simulink model "e5_3blocks_nn"  (R2020a)
settings: Solver=VariableStepAuto  StartTime=0.0  StopTime=10.0  RelTol=1e-3
undefined symbols (not defined in the file or in its folder): Quad
libraries: neural x123
(part 6 of 6)

== system e5_3blocks_nn/NN_online/Layer 3/Delays 1 ==
  "p{3}" : Inport  PortDimensions=30
      mask Display: e = 0.06;c1 = [120 230 180]/255;c2 = ([120 230 180]+0)/(256+128);c3 = ([120 230 180]+128)/(256+128);patch([0 1 1 0],[0 0 1 1],c1);patch([0 1 1 1-e 1-e 0+e],[0 0 1 1-e 0+e 0+e],c2);patch([0 0 1 1-e 0+e 0+e],[0 1 1 1-e 1-e 0+e],c3);plot([0 1 1 0 0],[0 0 1 1 0]);
  mux : Mux  Inputs=1
      mask Display: e = 0.06;c1 = [120 150 230]/255;c2 = ([120 150 230]+0)/383;c3 = ([120 150 230]+128)/383;patch([0 1 1 0],[0 0 1 1],c1);patch([0 1 1 1-e 1-e 0+e],[0 0 1 1-e 0+e 0+e],c2);patch([0 0 1 1-e 0+e 0+e],[0 1 1 1-e 1-e 0+e],c3);plot([0 1 1 0 0],[0 0 1 1 0]);disp('Mux')
  "pd{3,2}" : Outport
      mask Display: e = 0.06;c1 = [120 230 180]/255;c2 = ([120 230 180]+0)/(256+128);c3 = ([120 230 180]+128)/(256+128);patch([0 1 1 0],[0 0 1 1],c1);patch([0 1 1 1-e 1-e 0+e],[0 0 1 1-e 0+e 0+e],c2);patch([0 0 1 1-e 0+e 0+e],[0 1 1 1-e 1-e 0+e],c3);plot([0 1 1 0 0],[0 0 1 1 0]);
  wires:
  "p{3}"/1 -> mux/1
  mux/1 -> "pd{3,2}"/1

== system e5_3blocks_nn/NN_online/Layer 3/LW{3,2} ==
  "ad{3,2}" : Inport  PortDimensions=30
      mask Display: e = 0.06;c1 = [120 230 180]/255;c2 = ([120 230 180]+0)/(256+128);c3 = ([120 230 180]+128)/(256+128);patch([0 1 1 0],[0 0 1 1],c1);patch([0 1 1 1-e 1-e 0+e],[0 0 1 1-e 0+e 0+e],c2);patch([0 0 1 1-e 0+e 0+e],[0 1 1 1-e 1-e 0+e],c3);plot([0 1 1 0 0],[0 0 1 1 0]);
  "IW{3,2}(1,:)'" : Constant  Value=[-0.74045949711400804726935120925190858542919158935546875;-0.58401602771112093304139989413670264184474945068359375;-0.6034755109337701650673579933936707675457000732421875;0.269375496708191108918839518082677386701107025146484375;0.98280475536531586300270646461285650730133056640625;0.75298003196986418306124733135220594704151153564453125;0.0651266582356064549497176585646229796111583709716796875;-0.1734064841429667769290290380013175308704376220703125;0.45505253649777677171783807352767325937747955322265625;-1.1110777342299797965097241103649139404296875;-0.414174790218542920872124568631988950073719024658203125;1.2941375398693637510660892075975425541400909423828125;-0.255150133567479453500226327378186397254467010498046875;-1.5350351214048298942316250759176909923553466796875;0.309272282263894193743425375942024402320384979248046875;0.79832303482539657135674815435777418315410614013671875;-0.21477532944557797822682232435909099876880645751953125;0.294688422156485885228249799183686263859272003173828125;-0.4815517552196044714918343743192963302135467529296875;0.95724738920766172523002524030744098126888275146484375;-0.90955459212049583062054125548456795513629913330078125;0.346384843600047676037689825534471310675144195556640625;1.8649580259717961627785598466289229691028594970703125;0.80254294735749820421943923065555281937122344970703125;-0.03189069800816642097363029506595921702682971954345703125;0.88260884721326393620444150656112469732761383056640625;0.7140768958629133411619704929762519896030426025390625;-0.7406443636227937332705550943501293659210205078125;1.04882730776492483215633910731412470340728759765625;-0.468039530733766195869094417503220029175281524658203125]
      mask Display: e = 0.06;c1 = [120 150 230]/255;c2 = ([120 150 230]+0)/383;c3 = ([120 150 230]+128)/383;patch([0 1 1 0],[0 0 1 1],c1);patch([0 1 1 1-e 1-e 0+e],[0 0 1 1-e 0+e 0+e],c2);patch([0 0 1 1-e 0+e 0+e],[0 1 1 1-e 1-e 0+e],c3);plot([0 1 1 0 0],[0 0 1 1 0]);disp('weights');
  "IW{3,2}(2,:)'" : Constant  Value=[0.90649377307499701128534752569976262748241424560546875;-1.0137112713112188533415292113204486668109893798828125;0.329266995171617171678235536091960966587066650390625;0.2272975460759009413980180625003413297235965728759765625;0.50483842467994100022821157836006022989749908447265625;-0.27847685276827949252265170798636972904205322265625;-0.6308411790373049665703319988097064197063446044921875;-0.92392844182607591907441246803500689566135406494140625;0.429078778776798286376248370288521982729434967041015625;-0.85715776869411997029857275265385396778583526611328125;-1.0331789389061454276230733739794231951236724853515625;1.0713717274822391889443906620726920664310455322265625;-0.962090121894081828912703713285736739635467529296875;1.437254550428958221885977764031849801540374755859375;1.0336640551385924968741392149240709841251373291015625;0.5236554999268692167646577217965386807918548583984375;-1.1230558973221371754647179841413162648677825927734375;1.045419667606716895846830084337852895259857177734375;0.90531647821300020861912116743042133748531341552734375;0.8699142566681159483010787880630232393741607666015625;-0.2165646035040668937465824228638666681945323944091796875;0.9203162175351156104596839213627390563488006591796875;-0.47115506813383489781443813626538030803203582763671875;0.429130371212704642136515076344949193298816680908203125;-0.2803733814934059598300564175588078796863555908203125;-0.380720228824799333811057522325427271425724029541015625;0.263655099975223683461678092498914338648319244384765625;-0.68403898271574858913623984335572458803653717041015625;0.78282470489094857502010427197092212736606597900390625;0.53510283155604898563950655443477444350719451904296875]
      mask Display: e = 0.06;c1 = [120 150 230]/255;c2 = ([120 150 230]+0)/383;c3 = ([120 150 230]+128)/383;patch([0 1 1 0],[0 0 1 1],c1);patch([0 1 1 1-e 1-e 0+e],[0 0 1 1-e 0+e 0+e],c2);patch([0 0 1 1-e 0+e 0+e],[0 1 1 1-e 1-e 0+e],c3);plot([0 1 1 0 0],[0 0 1 1 0]);disp('weights');
  Mux : Mux  Inputs=2
      mask Display: e = 0.06;c1 = [120 150 230]/255;c2 = ([120 150 230]+0)/383;c3 = ([120 150 230]+128)/383;patch([0 1 1 0],[0 0 1 1],c1);patch([0 1 1 1-e 1-e 0+e],[0 0 1 1-e 0+e 0+e],c2);patch([0 0 1 1-e 0+e 0+e],[0 1 1 1-e 1-e 0+e],c3);plot([0 1 1 0 0],[0 0 1 1 0]);disp('Mux');
  dotprod1 : neural/Weight Functions/dotprod
  dotprod2 : neural/Weight Functions/dotprod
  "lz{3,2}" : Outport
      mask Display: e = 0.06;c1 = [120 230 180]/255;c2 = ([120 230 180]+0)/(256+128);c3 = ([120 230 180]+128)/(256+128);patch([0 1 1 0],[0 0 1 1],c1);patch([0 1 1 1-e 1-e 0+e],[0 0 1 1-e 0+e 0+e],c2);patch([0 0 1 1-e 0+e 0+e],[0 1 1 1-e 1-e 0+e],c3);plot([0 1 1 0 0],[0 0 1 1 0]);
  wires:
  "IW{3,2}(1,:)'"/1 -> dotprod1/1
  "ad{3,2}"/1 -> dotprod1/2, dotprod2/2
  dotprod1/1 -> Mux/1
  "IW{3,2}(2,:)'"/1 -> dotprod2/1
  dotprod2/1 -> Mux/2
  Mux/1 -> "lz{3,2}"/1
